simulink model "SPGF_FSK_0000_R2022b"  (R2022b)
settings: Solver=ode4  StartTime=0.0  StopTime=1.4  FixedStep=50e-6/50  RelTol=1e-3  EnableMultiTasking=on
undefined symbols (not defined in the file): D11, Delta
libraries: spsSeriesRLCBranchLib x1646, spsGroundLib x360, spsStairGeneratorLib x147, spsIdealSwitchLib x145, spsCurrentMeasurementLib x145, spsUniversalBridgeLib x76, spsThreePhaseSeriesRLCLoadLib x57, simulink x45, spsBistableLib x36, spsSequenceAnalyzerLib x31, spsThreePhaseParallelRLCLoadLib x20, spsThreePhaseTransformerTwoWindingsLib x20
(part 6 of 40)

== system SPGF_FSK_0000_R2022b/TP42 ==
  Load : spsThreePhaseParallelRLCLoadLib/Three-Phase Parallel RLC Load  Commented=on  LConnTagsString=A|B|C  Configuration=Y (grounded)  NominalVoltage=380  Vabc=[1e3 1e3 1e3]  Vabcp=[1e3 1e3 1e3]  NominalFrequency=50  UnbalancedPower=off  ActivePower=352800  InductivePower=158760  CapacitivePower=0  Pabc=[10e3 9e3 11e3]  QLabc=[100 90 110]  QCabc=[100 90 110]  Pabcp=[10e3 9e3 11e3]  QLabcp=[100 90 110]  QCabcp=[100 90 110]  Measurements=None  LoadType=constant PQ
  Nonlinear Load : Subsystem  Commented=on
  Nonlinear Load 3ph : Subsystem
  Q : Subsystem
  T : spsThreePhaseTransformerTwoWindingsLib/Three-Phase Transformer (Two Windings)  Winding1Connection=Delta (D11)  Winding2Connection=Yg  CoreType=Three single-phase transformers  SetSaturation=on  Hysteresis=off  DataFile='hysteresis'  SetInitialFlux=off  Measurements=None  UNITS=pu  NominalPower=[630000, 50]  Winding1=[10250, 0.00603175, 0.02750000]  Winding2=[400.00, 0.00603175, 0.02750000]  Rm=504  Lm=58.8235  L0=2  Saturation=[0 0;0.01774 0.324129;0.0487637 0.61284;0.0980856 0.825118;0.2 1;0.309543 1.08024;0.652348 1.17344;2.0357 1.26115;6.0215 1.36094;12.4388 1.49469]  InitialFluxes=[0.547022493837308 0.502268865215099 -1.04929135905267]  BreakLoop=on  DiscreteSolver=Trapezoidal iterative  DataType=off  TransfoNumber=1
  Three-Phase Series RLC Load : spsThreePhaseSeriesRLCLoadLib/Three-Phase Series RLC Load  Commented=on  LConnTagsString=A|B|C  Configuration=Y (grounded)  NominalVoltage=380  Vabc=[1e3 1e3 1e3]  Vabcp=[1e3 1e3 1e3]  NominalFrequency=50  UnbalancedPower=off  ActivePower=352800  InductivePower=158760  CapacitivePower=0  Pabc=[10e3 9e3 11e3]  QLabc=[100 90 110]  QCabc=[100 90 110]  Pabcp=[10e3 9e3 11e3]  QLabcp=[100 90 110]  QCabcp=[100 90 110]  Measurements=None  LoadType=constant Z
  Three-Phase Series RLC Load1 : spsThreePhaseSeriesRLCLoadLib/Three-Phase Series RLC Load  LConnTagsString=A|B|C  Configuration=Y (grounded)  NominalVoltage=380  Vabc=[1e3 1e3 1e3]  Vabcp=[1e3 1e3 1e3]  NominalFrequency=50  UnbalancedPower=off  ActivePower=0.1*352800  InductivePower=0  CapacitivePower=0  Pabc=[10e3 9e3 11e3]  QLabc=[100 90 110]  QCabc=[100 90 110]  Pabcp=[10e3 9e3 11e3]  QLabcp=[100 90 110]  QCabcp=[100 90 110]  Measurements=None  LoadType=constant Z
  Three-Phase Series RLC Load2 : spsThreePhaseSeriesRLCLoadLib/Three-Phase Series RLC Load  LConnTagsString=A|B|C  Configuration=Y (grounded)  NominalVoltage=380  Vabc=[1e3 1e3 1e3]  Vabcp=[1e3 1e3 1e3]  NominalFrequency=50  UnbalancedPower=off  ActivePower=0.9*352800  InductivePower=158760  CapacitivePower=0  Pabc=[10e3 9e3 11e3]  QLabc=[100 90 110]  QCabc=[100 90 110]  Pabcp=[10e3 9e3 11e3]  QLabcp=[100 90 110]  QCabcp=[100 90 110]  Measurements=None  LoadType=constant Z
  A : PMIOPort  Side=Right
  B : PMIOPort  Port=2  Side=Right
  C : PMIOPort  Port=3  Side=Right
  connections:
  Q/LConn3 -- T/LConn3
  Q/LConn1 -- T/LConn1
  Q/RConn2 -- B/RConn1
  Q/RConn1 -- A/RConn1
  Q/LConn2 -- T/LConn2
  Q/RConn3 -- C/RConn1
  Three-Phase Series RLC Load1/LConn3 -- Three-Phase Series RLC Load2/LConn3 -- Three-Phase Series RLC Load/LConn3 -- Nonlinear Load/LConn3 -- Nonlinear Load 3ph/LConn3 -- T/RConn3 -- Load/LConn3
  Three-Phase Series RLC Load1/LConn2 -- Three-Phase Series RLC Load2/LConn2 -- Three-Phase Series RLC Load/LConn2 -- Nonlinear Load/LConn2 -- Nonlinear Load 3ph/LConn2 -- Load/LConn2 -- T/RConn2
  Three-Phase Series RLC Load2/LConn1 -- Three-Phase Series RLC Load1/LConn1 -- Three-Phase Series RLC Load/LConn1 -- Nonlinear Load/LConn1 -- Nonlinear Load 3ph/LConn1 -- Load/LConn1 -- T/RConn1

== system SPGF_FSK_0000_R2022b/TP43 ==
  Load : spsThreePhaseParallelRLCLoadLib/Three-Phase Parallel RLC Load  Commented=on  LConnTagsString=A|B|C  Configuration=Y (grounded)  NominalVoltage=380  Vabc=[1e3 1e3 1e3]  Vabcp=[1e3 1e3 1e3]  NominalFrequency=50  UnbalancedPower=off  ActivePower=224000  InductivePower=100800  CapacitivePower=0  Pabc=[10e3 9e3 11e3]  QLabc=[100 90 110]  QCabc=[100 90 110]  Pabcp=[10e3 9e3 11e3]  QLabcp=[100 90 110]  QCabcp=[100 90 110]  Measurements=None  LoadType=constant PQ
  Nonlinear Load : Subsystem  Commented=on
  Nonlinear Load 3ph : Subsystem
  Q : Subsystem
  T : spsThreePhaseTransformerTwoWindingsLib/Three-Phase Transformer (Two Windings)  Winding1Connection=Y  Winding2Connection=Yg  CoreType=Three single-phase transformers  SetSaturation=on  Hysteresis=off  DataFile='hysteresis'  SetInitialFlux=off  Measurements=None  UNITS=pu  NominalPower=[400000, 50]  Winding1=[10250, 0.00687500, 0.02250000]  Winding2=[400.00, 0.00687500, 0.02250000]  Rm=444.444  Lm=55.5556  L0=2  Saturation=[0 0;0.01774 0.324129;0.0487637 0.61284;0.0980856 0.825118;0.2 1;0.309543 1.08024;0.652348 1.17344;2.0357 1.26115;6.0215 1.36094;12.4388 1.49469]  InitialFluxes=[0.0224556996451499 0.89821690421441 -0.920672603859515]  BreakLoop=on  DiscreteSolver=Trapezoidal iterative  DataType=off  TransfoNumber=1
  Three-Phase Series RLC Load : spsThreePhaseSeriesRLCLoadLib/Three-Phase Series RLC Load  Commented=on  LConnTagsString=A|B|C  Configuration=Y (grounded)  NominalVoltage=380  Vabc=[1e3 1e3 1e3]  Vabcp=[1e3 1e3 1e3]  NominalFrequency=50  UnbalancedPower=off  ActivePower=224000  InductivePower=100800  CapacitivePower=0  Pabc=[10e3 9e3 11e3]  QLabc=[100 90 110]  QCabc=[100 90 110]  Pabcp=[10e3 9e3 11e3]  QLabcp=[100 90 110]  QCabcp=[100 90 110]  Measurements=None  LoadType=constant Z
  Three-Phase Series RLC Load1 : spsThreePhaseSeriesRLCLoadLib/Three-Phase Series RLC Load  LConnTagsString=A|B|C  Configuration=Y (grounded)  NominalVoltage=380  Vabc=[1e3 1e3 1e3]  Vabcp=[1e3 1e3 1e3]  NominalFrequency=50  UnbalancedPower=off  ActivePower=0.1*224000  InductivePower=0  CapacitivePower=0  Pabc=[10e3 9e3 11e3]  QLabc=[100 90 110]  QCabc=[100 90 110]  Pabcp=[10e3 9e3 11e3]  QLabcp=[100 90 110]  QCabcp=[100 90 110]  Measurements=None  LoadType=constant Z
  Three-Phase Series RLC Load2 : spsThreePhaseSeriesRLCLoadLib/Three-Phase Series RLC Load  LConnTagsString=A|B|C  Configuration=Y (grounded)  NominalVoltage=380  Vabc=[1e3 1e3 1e3]  Vabcp=[1e3 1e3 1e3]  NominalFrequency=50  UnbalancedPower=off  ActivePower=0.9*224000  InductivePower=100800  CapacitivePower=0  Pabc=[10e3 9e3 11e3]  QLabc=[100 90 110]  QCabc=[100 90 110]  Pabcp=[10e3 9e3 11e3]  QLabcp=[100 90 110]  QCabcp=[100 90 110]  Measurements=None  LoadType=constant Z
  A : PMIOPort  Side=Right
  B : PMIOPort  Port=2  Side=Right
  C : PMIOPort  Port=3  Side=Right
  connections:
  Three-Phase Series RLC Load2/LConn1 -- Three-Phase Series RLC Load1/LConn1 -- Three-Phase Series RLC Load/LConn1 -- Nonlinear Load/LConn1 -- Nonlinear Load 3ph/LConn1 -- Load/LConn1 -- T/RConn1
  Three-Phase Series RLC Load2/LConn2 -- Three-Phase Series RLC Load1/LConn2 -- Three-Phase Series RLC Load/LConn2 -- Nonlinear Load/LConn2 -- Nonlinear Load 3ph/LConn2 -- Load/LConn2 -- T/RConn2
  Three-Phase Series RLC Load2/LConn3 -- Three-Phase Series RLC Load1/LConn3 -- Three-Phase Series RLC Load/LConn3 -- Nonlinear Load/LConn3 -- Nonlinear Load 3ph/LConn3 -- T/RConn3 -- Load/LConn3
  Q/RConn3 -- C/RConn1
  Q/LConn2 -- T/LConn2
  Q/RConn1 -- A/RConn1
  Q/RConn2 -- B/RConn1
  Q/LConn1 -- T/LConn1
  Q/LConn3 -- T/LConn3

== system SPGF_FSK_0000_R2022b/TP51 ==
  Load : spsThreePhaseParallelRLCLoadLib/Three-Phase Parallel RLC Load  Commented=on  LConnTagsString=A|B|C  Configuration=Y (grounded)  NominalVoltage=380  Vabc=[1e3 1e3 1e3]  Vabcp=[1e3 1e3 1e3]  NominalFrequency=50  UnbalancedPower=off  ActivePower=224000  InductivePower=100800  CapacitivePower=0  Pabc=[10e3 9e3 11e3]  QLabc=[100 90 110]  QCabc=[100 90 110]  Pabcp=[10e3 9e3 11e3]  QLabcp=[100 90 110]  QCabcp=[100 90 110]  Measurements=None  LoadType=constant PQ
  Nonlinear Load : Subsystem  Commented=on
  Nonlinear Load 3ph : Subsystem
  Q : Subsystem
  T : spsThreePhaseTransformerTwoWindingsLib/Three-Phase Transformer (Two Windings)  Winding1Connection=Y  Winding2Connection=Yg  CoreType=Three single-phase transformers  SetSaturation=on  Hysteresis=off  DataFile='hysteresis'  SetInitialFlux=off  Measurements=None  UNITS=pu  NominalPower=[400000, 50]  Winding1=[10250, 0.00687500, 0.02250000]  Winding2=[400.00, 0.00687500, 0.02250000]  Rm=444.444  Lm=55.5556  L0=2  Saturation=[0 0;0.01774 0.324129;0.0487637 0.61284;0.0980856 0.825118;0.2 1;0.309543 1.08024;0.652348 1.17344;2.0357 1.26115;6.0215 1.36094;12.4388 1.49469]  InitialFluxes=[0.0226319899806227 0.898092550893289 -0.920724540873739]  BreakLoop=on  DiscreteSolver=Trapezoidal iterative  DataType=off  TransfoNumber=1
  Three-Phase Series RLC Load : spsThreePhaseSeriesRLCLoadLib/Three-Phase Series RLC Load  Commented=on  LConnTagsString=A|B|C  Configuration=Y (grounded)  NominalVoltage=380  Vabc=[1e3 1e3 1e3]  Vabcp=[1e3 1e3 1e3]  NominalFrequency=50  UnbalancedPower=off  ActivePower=224000  InductivePower=100800  CapacitivePower=0  Pabc=[10e3 9e3 11e3]  QLabc=[100 90 110]  QCabc=[100 90 110]  Pabcp=[10e3 9e3 11e3]  QLabcp=[100 90 110]  QCabcp=[100 90 110]  Measurements=None  LoadType=constant Z
  Three-Phase Series RLC Load1 : spsThreePhaseSeriesRLCLoadLib/Three-Phase Series RLC Load  LConnTagsString=A|B|C  Configuration=Y (grounded)  NominalVoltage=380  Vabc=[1e3 1e3 1e3]  Vabcp=[1e3 1e3 1e3]  NominalFrequency=50  UnbalancedPower=off  ActivePower=0.1*224000  InductivePower=0  CapacitivePower=0  Pabc=[10e3 9e3 11e3]  QLabc=[100 90 110]  QCabc=[100 90 110]  Pabcp=[10e3 9e3 11e3]  QLabcp=[100 90 110]  QCabcp=[100 90 110]  Measurements=None  LoadType=constant Z
  Three-Phase Series RLC Load2 : spsThreePhaseSeriesRLCLoadLib/Three-Phase Series RLC Load  LConnTagsString=A|B|C  Configuration=Y (grounded)  NominalVoltage=380  Vabc=[1e3 1e3 1e3]  Vabcp=[1e3 1e3 1e3]  NominalFrequency=50  UnbalancedPower=off  ActivePower=0.9*224000  InductivePower=100800  CapacitivePower=0  Pabc=[10e3 9e3 11e3]  QLabc=[100 90 110]  QCabc=[100 90 110]  Pabcp=[10e3 9e3 11e3]  QLabcp=[100 90 110]  QCabcp=[100 90 110]  Measurements=None  LoadType=constant Z
  A : PMIOPort  Side=Right
  B : PMIOPort  Port=2  Side=Right
  C : PMIOPort  Port=3  Side=Right
  connections:
  Three-Phase Series RLC Load2/LConn1 -- Three-Phase Series RLC Load1/LConn1 -- Three-Phase Series RLC Load/LConn1 -- Nonlinear Load/LConn1 -- Nonlinear Load 3ph/LConn1 -- Load/LConn1 -- T/RConn1
  Three-Phase Series RLC Load2/LConn2 -- Three-Phase Series RLC Load1/LConn2 -- Three-Phase Series RLC Load/LConn2 -- Nonlinear Load/LConn2 -- Nonlinear Load 3ph/LConn2 -- Load/LConn2 -- T/RConn2
  Three-Phase Series RLC Load1/LConn3 -- Three-Phase Series RLC Load2/LConn3 -- Three-Phase Series RLC Load/LConn3 -- Nonlinear Load/LConn3 -- Nonlinear Load 3ph/LConn3 -- T/RConn3 -- Load/LConn3
  Q/RConn3 -- C/RConn1
  Q/LConn2 -- T/LConn2
  Q/RConn1 -- A/RConn1
  Q/RConn2 -- B/RConn1
  Q/LConn1 -- T/LConn1
  Q/LConn3 -- T/LConn3

== system SPGF_FSK_0000_R2022b/TP52 ==
  Load : spsThreePhaseParallelRLCLoadLib/Three-Phase Parallel RLC Load  Commented=on  LConnTagsString=A|B|C  Configuration=Y (grounded)  NominalVoltage=380  Vabc=[1e3 1e3 1e3]  Vabcp=[1e3 1e3 1e3]  NominalFrequency=50  UnbalancedPower=off  ActivePower=560000  InductivePower=252000  CapacitivePower=0  Pabc=[10e3 9e3 11e3]  QLabc=[100 90 110]  QCabc=[100 90 110]  Pabcp=[10e3 9e3 11e3]  QLabcp=[100 90 110]  QCabcp=[100 90 110]  Measurements=None  LoadType=constant PQ
  Nonlinear Load : Subsystem  Commented=on
  Nonlinear Load 3ph : Subsystem
  Q : Subsystem
  T : spsThreePhaseTransformerTwoWindingsLib/Three-Phase Transformer (Two Windings)  Winding1Connection=Y  Winding2Connection=Yg  CoreType=Three single-phase transformers  SetSaturation=on  Hysteresis=off  DataFile='hysteresis'  SetInitialFlux=off  Measurements=None  UNITS=pu  NominalPower=[1000000, 50]  Winding1=[10250, 0.00610000, 0.02750000]  Winding2=[400.00, 0.00610000, 0.02750000]  Rm=526.316  Lm=58.8235  L0=2  Saturation=[0 0;0.01774 0.324129;0.0487637 0.61284;0.0980856 0.825118;0.2 1;0.309543 1.08024;0.652348 1.17344;2.0357 1.26115;6.0215 1.36094;12.4388 1.49469]  InitialFluxes=[0.0255116004445126 0.893899314027236 -0.919410914471723]  BreakLoop=on  DiscreteSolver=Trapezoidal iterative  DataType=off  TransfoNumber=1
  Three-Phase Series RLC Load : spsThreePhaseSeriesRLCLoadLib/Three-Phase Series RLC Load  Commented=on  LConnTagsString=A|B|C  Configuration=Y (grounded)  NominalVoltage=380  Vabc=[1e3 1e3 1e3]  Vabcp=[1e3 1e3 1e3]  NominalFrequency=50  UnbalancedPower=off  ActivePower=560000  InductivePower=252000  CapacitivePower=0  Pabc=[10e3 9e3 11e3]  QLabc=[100 90 110]  QCabc=[100 90 110]  Pabcp=[10e3 9e3 11e3]  QLabcp=[100 90 110]  QCabcp=[100 90 110]  Measurements=None  LoadType=constant Z
  Three-Phase Series RLC Load1 : spsThreePhaseSeriesRLCLoadLib/Three-Phase Series RLC Load  LConnTagsString=A|B|C  Configuration=Y (grounded)  NominalVoltage=380  Vabc=[1e3 1e3 1e3]  Vabcp=[1e3 1e3 1e3]  NominalFrequency=50  UnbalancedPower=off  ActivePower=0.1*560000  InductivePower=0  CapacitivePower=0  Pabc=[10e3 9e3 11e3]  QLabc=[100 90 110]  QCabc=[100 90 110]  Pabcp=[10e3 9e3 11e3]  QLabcp=[100 90 110]  QCabcp=[100 90 110]  Measurements=None  LoadType=constant Z
  Three-Phase Series RLC Load2 : spsThreePhaseSeriesRLCLoadLib/Three-Phase Series RLC Load  LConnTagsString=A|B|C  Configuration=Y (grounded)  NominalVoltage=380  Vabc=[1e3 1e3 1e3]  Vabcp=[1e3 1e3 1e3]  NominalFrequency=50  UnbalancedPower=off  ActivePower=0.9*560000  InductivePower=252000  CapacitivePower=0  Pabc=[10e3 9e3 11e3]  QLabc=[100 90 110]  QCabc=[100 90 110]  Pabcp=[10e3 9e3 11e3]  QLabcp=[100 90 110]  QCabcp=[100 90 110]  Measurements=None  LoadType=constant Z
  A : PMIOPort  Side=Right
  B : PMIOPort  Port=2  Side=Right
  C : PMIOPort  Port=3  Side=Right
  connections:
  Q/LConn3 -- T/LConn3
  Q/LConn1 -- T/LConn1
  Q/RConn2 -- B/RConn1
  Q/RConn1 -- A/RConn1
  Q/LConn2 -- T/LConn2
  Q/RConn3 -- C/RConn1
  Three-Phase Series RLC Load1/LConn3 -- Three-Phase Series RLC Load2/LConn3 -- Nonlinear Load/LConn3 -- Nonlinear Load 3ph/LConn3 -- T/RConn3 -- Load/LConn3 -- Three-Phase Series RLC Load/LConn3
  Three-Phase Series RLC Load1/LConn2 -- Three-Phase Series RLC Load2/LConn2 -- Nonlinear Load/LConn2 -- Nonlinear Load 3ph/LConn2 -- Load/LConn2 -- T/RConn2 -- Three-Phase Series RLC Load/LConn2
  Three-Phase Series RLC Load/LConn1 -- Nonlinear Load/LConn1 -- Nonlinear Load 3ph/LConn1 -- T/RConn1 -- Load/LConn1 -- Three-Phase Series RLC Load2/LConn1 -- Three-Phase Series RLC Load1/LConn1

== system SPGF_FSK_0000_R2022b/TP53 ==
  Load : spsThreePhaseParallelRLCLoadLib/Three-Phase Parallel RLC Load  Commented=on  LConnTagsString=A|B|C  Configuration=Y (grounded)  NominalVoltage=380  Vabc=[1e3 1e3 1e3]  Vabcp=[1e3 1e3 1e3]  NominalFrequency=50  UnbalancedPower=off  ActivePower=224000  InductivePower=100800  CapacitivePower=0  Pabc=[10e3 9e3 11e3]  QLabc=[100 90 110]  QCabc=[100 90 110]  Pabcp=[10e3 9e3 11e3]  QLabcp=[100 90 110]  QCabcp=[100 90 110]  Measurements=None  LoadType=constant PQ
  Nonlinear Load : Subsystem  Commented=on
  Nonlinear Load 3ph : Subsystem
  Q : Subsystem
  T : spsThreePhaseTransformerTwoWindingsLib/Three-Phase Transformer (Two Windings)  Winding1Connection=Y  Winding2Connection=Yg  CoreType=Three single-phase transformers  SetSaturation=on  Hysteresis=off  DataFile='hysteresis'  SetInitialFlux=off  Measurements=None  UNITS=pu  NominalPower=[400000, 50]  Winding1=[10250, 0.00687500, 0.02250000]  Winding2=[400.00, 0.00687500, 0.02250000]  Rm=444.444  Lm=55.5556  L0=2  Saturation=[0 0;0.01774 0.324129;0.0487637 0.61284;0.0980856 0.825118;0.2 1;0.309543 1.08024;0.652348 1.17344;2.0357 1.26115;6.0215 1.36094;12.4388 1.49469]  InitialFluxes=[0.0221773071271057 0.896403452288866 -0.918580759415872]  BreakLoop=on  DiscreteSolver=Trapezoidal iterative  DataType=off  TransfoNumber=1
  Three-Phase Series RLC Load : spsThreePhaseSeriesRLCLoadLib/Three-Phase Series RLC Load  Commented=on  LConnTagsString=A|B|C  Configuration=Y (grounded)  NominalVoltage=380  Vabc=[1e3 1e3 1e3]  Vabcp=[1e3 1e3 1e3]  NominalFrequency=50  UnbalancedPower=off  ActivePower=224000  InductivePower=100800  CapacitivePower=0  Pabc=[10e3 9e3 11e3]  QLabc=[100 90 110]  QCabc=[100 90 110]  Pabcp=[10e3 9e3 11e3]  QLabcp=[100 90 110]  QCabcp=[100 90 110]  Measurements=None  LoadType=constant Z
  Three-Phase Series RLC Load1 : spsThreePhaseSeriesRLCLoadLib/Three-Phase Series RLC Load  LConnTagsString=A|B|C  Configuration=Y (grounded)  NominalVoltage=380  Vabc=[1e3 1e3 1e3]  Vabcp=[1e3 1e3 1e3]  NominalFrequency=50  UnbalancedPower=off  ActivePower=0.1*224000  InductivePower=0  CapacitivePower=0  Pabc=[10e3 9e3 11e3]  QLabc=[100 90 110]  QCabc=[100 90 110]  Pabcp=[10e3 9e3 11e3]  QLabcp=[100 90 110]  QCabcp=[100 90 110]  Measurements=None  LoadType=constant Z
  Three-Phase Series RLC Load2 : spsThreePhaseSeriesRLCLoadLib/Three-Phase Series RLC Load  LConnTagsString=A|B|C  Configuration=Y (grounded)  NominalVoltage=380  Vabc=[1e3 1e3 1e3]  Vabcp=[1e3 1e3 1e3]  NominalFrequency=50  UnbalancedPower=off  ActivePower=0.9*224000  InductivePower=100800  CapacitivePower=0  Pabc=[10e3 9e3 11e3]  QLabc=[100 90 110]  QCabc=[100 90 110]  Pabcp=[10e3 9e3 11e3]  QLabcp=[100 90 110]  QCabcp=[100 90 110]  Measurements=None  LoadType=constant Z
  A : PMIOPort  Side=Right
  B : PMIOPort  Port=2  Side=Right
  C : PMIOPort  Port=3  Side=Right
  connections:
  Three-Phase Series RLC Load1/LConn1 -- Three-Phase Series RLC Load2/LConn1 -- Three-Phase Series RLC Load/LConn1 -- Nonlinear Load/LConn1 -- Nonlinear Load 3ph/LConn1 -- T/RConn1 -- Load/LConn1
  Three-Phase Series RLC Load2/LConn2 -- Three-Phase Series RLC Load1/LConn2 -- Three-Phase Series RLC Load/LConn2 -- Nonlinear Load/LConn2 -- Nonlinear Load 3ph/LConn2 -- T/RConn2 -- Load/LConn2
  Three-Phase Series RLC Load2/LConn3 -- Three-Phase Series RLC Load1/LConn3 -- Three-Phase Series RLC Load/LConn3 -- Nonlinear Load/LConn3 -- Nonlinear Load 3ph/LConn3 -- T/RConn3 -- Load/LConn3
  Q/RConn3 -- C/RConn1
  Q/LConn2 -- T/LConn2
  Q/RConn1 -- A/RConn1
  Q/RConn2 -- B/RConn1
  Q/LConn1 -- T/LConn1
  Q/LConn3 -- T/LConn3

== system SPGF_FSK_0000_R2022b/TSN ==
  DGR : Subsystem  Commented=on  mask{Freq=50, Current=19.26, CompFactor=0, Voltage=6090, Lt=0.0091667, TangLoss=0.02}
      mask prompts: Freq "Frequency, [Hz]"; Current "Compensated Current, [A]"; CompFactor "Compensation Factor, [-0.2,..., 0.2]"; Voltage "Voltage at DGR"; Lt "Transformer inductance [ L1(H)]"; TangLoss "Loss factor"
      mask init:
      | % L = 1350e-3;
      | Icomp = -(CompFactor*Current-Current);
      | L = (Voltage/Icomp)/(2*pi*Freq)-Lt;
      | Rm = 2*pi*Freq*L*TangLoss/2;
      | Rst = ((2*pi*Freq*L)^2+Rm^2)/Rm;
  Ground1 : spsGroundLib/Ground  Commented=on  LConnTagsString=a
  Rst : spsSeriesRLCBranchLib/Series RLC Branch  Commented=on  LConnTagsString=__new0  RConnTagsString=__new0  BranchType=R  Resistance=100  Inductance=1000e-3  SetiL0=off  InitialCurrent=0  Capacitance=1e-6  Setx0=off  InitialVoltage=0  Measurements=None
  TSN : spsThreePhaseTransformerTwoWindingsLib/Three-Phase Transformer (Two Windings)  Winding1Connection=Yn  Winding2Connection=Delta (D11)  CoreType=Three single-phase transformers  SetSaturation=on  Hysteresis=off  DataFile='hysteresis'  SetInitialFlux=off  Measurements=None  UNITS=pu  NominalPower=[250000 50]  Winding1=[10250 0.0076 0.0275]  Winding2=[400 0.0076 0.0275]  Rm=249.99  Lm=28.571  L0=0.66885  Saturation=[0 0;0.0010988 0.1;0.0024217 0.2;0.0040219 0.3;0.0059961 0.40001;0.0084933 0.50001;0.011751 0.60001;0.016177 0.70001;0.022532 0.80001;0.032408 0.90001;0.049756 1;0.087393 1.1;0.20927 1.2;0.70928 1.3;1.5874 1.4;2.5497 1.5]  InitialFluxes=[0.0107246931876914 0.916304027052604 -0.927028720240254]  BreakLoop=on  DiscreteSolver=Trapezoidal iterative  DataType=off  TransfoNumber=1
  A : PMIOPort  Side=Left
  B : PMIOPort  Port=2  Side=Left
  C : PMIOPort  Port=3  Side=Left
  connections:
  TSN/LConn1 -- A/RConn1
  TSN/LConn3 -- C/RConn1
  TSN/LConn2 -- B/RConn1
  DGR/RConn1 -- Rst/RConn1 -- TSN/LConn4
  Ground1/LConn1 -- Rst/LConn1

== system SPGF_FSK_0000_R2022b/V1 ==
  Sum of Elements : Sum  Inputs=+
  Three-Phase V-I Measurement : spsThreePhaseVIMeasurementLib/Three-Phase V-I Measurement  VoltageMeasurement=phase-to-ground  SetLabelV=off  LabelV=Vabc  Vpu=off  VpuLL=off  CurrentMeasurement=no  SetLabelI=off  LabelI=Iabc  Ipu=off  Pbase=100e6  Vbase=500e3  OutputType=Complex  PhasorSimulation=off  PSBequivalent=0
  VT : Subsystem
  A : PMIOPort  Side=Left
  B : PMIOPort  Port=2  Side=Left
  C : PMIOPort  Port=3  Side=Left
  tag scope: M3U0_V1=global, M3U0_VT1=global, MUabc1_VT1=global, MUabc2_VT1=global, MUabc_V1=global
  wires:
  VT/1(Uabc1) -> [MUabc1_VT1]
  VT/2(Uabc2) -> [MUabc2_VT1]
  VT/3(3U0) -> [M3U0_VT1]
  Sum of Elements/1 -> [M3U0_V1]
  Three-Phase V-I Measurement/1 -> [MUabc_V1], Sum of Elements/1
  connections:
  VT/LConn2 -- Three-Phase V-I Measurement/LConn2 -- B/RConn1
  Three-Phase V-I Measurement/LConn1 -- VT/LConn1 -- A/RConn1
  C/RConn1 -- Three-Phase V-I Measurement/LConn3 -- VT/LConn3

== system SPGF_FSK_0000_R2022b/V53 ==
  VT : Subsystem
  A : PMIOPort  Side=Left
  B : PMIOPort  Port=2  Side=Left
  C : PMIOPort  Port=3  Side=Left
  tag scope: M3U0_VT53=global, MUabc1_VT53=global, MUabc2_VT53=global
  wires:
  VT/1(Uabc1) -> [MUabc1_VT53]
  VT/2(Uabc2) -> [MUabc2_VT53]
  VT/3(3U0) -> [M3U0_VT53]
  connections:
  VT/LConn2 -- B/RConn1
  VT/LConn1 -- A/RConn1
  VT/LConn3 -- C/RConn1

== system SPGF_FSK_0000_R2022b/W11 ==
  DPL : Subsystem  Commented=on  mask{N=6, Frequency=[50], R_matrix=[0.16804171053251 0.0494303508468275 0.0494307138863892 0.0494307138863892 0.0494307138863892 0.0494307138863892;0.0494303508468275 0.453964608408466 0.0494307138863892 0.0494307138863892 0.0494307138863892 0.0494307138863892;0.0494307138863892 0.0494307138863892 0.168042542894219 0.0494311832085362 0.0494315463631826 0.0494315463631826;0.0494307138863892 0.0494307138863892 0.0494311832085362 0.453965440770175 0.0494315463631826 0.0494315463631826;0.0494307138863892 0.0494307138863892 0.0494315463631826 0.0494315463631826 0.168042542894219 0.0494311832085362;0.0494307138863892 0.0494307138863892 0.0494315463631826 0.0494315463631826 0.0494311832085362 0.453965440770175], L_matrix=[0.00251009633073536 0.00236486393083554 0.00216527915989806 0.00216527915989806 0.00216527915989806 0.00216527915989806;0.00236486393083554 0.00236372630589008 0.00216527915989806 0.00216527915989806 0.00216527915989806 0.00216527915989806;0.00216527915989806 0.00216527915989806 0.00243730728151529 0.00229207488161547 0.00218759083544916 0.00218759083544916;0.00216527915989806 0.00216527915989806 0.00229207488161547 0.00229093725667002 0.00218759083544916 0.00218759083544916;0.00216527915989806 0.00216527915989806 0.00218759083544916 0.00218759083544916 0.00243730728151529 0.00229207488161547;0.00216527915989806 0.00216527915989806 0.00218759083544916 0.00218759083544916 0.00229207488161547 0.00229093725667002], C_matrix=[2.72330746828679e-07 -2.72330746828679e-07 0 0 0 0;-2.72330746828679e-07 4.53349993591203e-07 0 0 0 0;0 0 2.72330746828679e-07 -2.72330746828679e-07 0 0;0 0 -2.72330746828679e-07 4.53349993591203e-07 0 0;0 0 0 0 2.72330746828679e-07 -2.72330746828679e-07;0 0 0 0 -2.72330746828679e-07 4.53349993591203e-07], Rg_matrix=[584417.826283929 -584417.826283929 Inf Inf Inf -Inf;-584417.826283929 351064.178541512 Inf Inf Inf -Inf;Inf Inf 584417.826283929 -584417.826283929 Inf -Inf;Inf Inf -584417.826283929 351064.178541512 Inf -Inf;Inf Inf Inf Inf 584417.826283929 -584417.826283929;Inf Inf Inf Inf -584417.826283929 351064.178541512], LineLength=[3]}
      mask prompts: N "Number of phases [N]"; Frequency "Frequency used for rlc specification [Hz]:"; R_matrix "Resistance per unit length [Ohms/km] NxN matrix"; L_matrix "Inductance per unit length [H/km] NxN matrix"; C_matrix "Capacitance per unit length [F/km] NxN matrix"; Rg_matrix "Resistance shunt matrix 6*6 [Ohm*km]"; LineLength "Line Length(km)"
      mask init:
      | % Rloss=1/(2*pi*Frequency*C_matrix(1,1)*TangLoss);
      | Rg_matrix=Rg_matrix./LineLength;
      mask Display:
      | port_label('lconn',1,'A');
      | port_label('lconn',2,'B');
      | port_label('lconn',3,'C');
      | 
      | port_label('rconn',1,'a');
      | port_label('rconn',2,'b');
      | port_label('rconn',3,'c');
      | 
      | disp('1x240');
  Pi : Subsystem  mask{R0=0.125, X0=0.075, Cp0=0.46, tg=2, Frequency=[50], LineLength=[3]}
      mask prompts: R0 "Удельное активное сопротивление, Ом/км"; X0 "Удельное индуктивное сопротивление, Ом/км"; Cp0 "Удельная рабочая емкость, мкФ/км"; tg "Тангенс диэлектрических потерь, %"; Frequency "Частота сети, Гц"; LineLength "Длина линии, км"
      mask init:
      | R=R0*LineLength;
      | L=X0*LineLength/(2*pi*Frequency);
      | Cp=Cp0*LineLength*1e-6;
      | Cmf=0.1525*Cp;
      | Cfg=0.56*Cp;
      | tg_pu=tg/100;
      | 
      | Rmf=1/(Cmf*2*pi*Frequency*tg_pu);
      | Rfg=1/(Cfg*2*pi*Frequency*tg_pu);
      mask Display:
      | port_label('lconn',1,'A');
      | port_label('lconn',2,'B');
      | port_label('lconn',3,'C');
      | 
      | port_label('rconn',1,'a');
      | port_label('rconn',2,'b');
      | port_label('rconn',3,'c');
      | 
      | disp('1x240');
  Q : Subsystem
  concentrated : Subsystem  Commented=on  mask{N=6, Frequency=[50], R_matrix=[0.16804171053251 0.0494303508468275 0.0494307138863892 0.0494307138863892 0.0494307138863892 0.0494307138863892;0.0494303508468275 0.453964608408466 0.0494307138863892 0.0494307138863892 0.0494307138863892 0.0494307138863892;0.0494307138863892 0.0494307138863892 0.168042542894219 0.0494311832085362 0.0494315463631826 0.0494315463631826;0.0494307138863892 0.0494307138863892 0.0494311832085362 0.453965440770175 0.0494315463631826 0.0494315463631826;0.0494307138863892 0.0494307138863892 0.0494315463631826 0.0494315463631826 0.168042542894219 0.0494311832085362;0.0494307138863892 0.0494307138863892 0.0494315463631826 0.0494315463631826 0.0494311832085362 0.453965440770175], L_matrix=[0.00251009633073536 0.00236486393083554 0.00216527915989806 0.00216527915989806 0.00216527915989806 0.00216527915989806;0.00236486393083554 0.00236372630589008 0.00216527915989806 0.00216527915989806 0.00216527915989806 0.00216527915989806;0.00216527915989806 0.00216527915989806 0.00243730728151529 0.00229207488161547 0.00218759083544916 0.00218759083544916;0.00216527915989806 0.00216527915989806 0.00229207488161547 0.00229093725667002 0.00218759083544916 0.00218759083544916;0.00216527915989806 0.00216527915989806 0.00218759083544916 0.00218759083544916 0.00243730728151529 0.00229207488161547;0.00216527915989806 0.00216527915989806 0.00218759083544916 0.00218759083544916 0.00229207488161547 0.00229093725667002], C_matrix=[2.72330746828679e-07 -2.72330746828679e-07 0 0 0 0;-2.72330746828679e-07 4.53349993591203e-07 0 0 0 0;0 0 2.72330746828679e-07 -2.72330746828679e-07 0 0;0 0 -2.72330746828679e-07 4.53349993591203e-07 0 0;0 0 0 0 2.72330746828679e-07 -2.72330746828679e-07;0 0 0 0 -2.72330746828679e-07 4.53349993591203e-07], Rg_matrix=[584417.826283929 -584417.826283929 Inf Inf Inf -Inf;-584417.826283929 351064.178541512 Inf Inf Inf -Inf;Inf Inf 584417.826283929 -584417.826283929 Inf -Inf;Inf Inf -584417.826283929 351064.178541512 Inf -Inf;Inf Inf Inf Inf 584417.826283929 -584417.826283929;Inf Inf Inf Inf -584417.826283929 351064.178541512], LineLength=[3]}
      mask prompts: N "Number of phases [N]"; Frequency "Frequency [Hz]:"; R_matrix "Resistance matrix 6*6 [Ohm/km]"; L_matrix "Inductance matrix 6*6 [H/km]"; C_matrix "Capacitance matrix 6*6 [F/km]"; Rg_matrix "Resistance shunt matrix 6*6 [Ohm*km]"; LineLength "Line Length(km)"
      mask init:
      | R_matrix=R_matrix.*LineLength;
      | L_matrix=L_matrix.*LineLength;
      | C_matrix=C_matrix.*LineLength;
      | Rg_matrix=Rg_matrix./LineLength;
      | 
      | % Rloss=1/(2*pi*Frequency*C_matrix(1,1)*TangLoss);
      | % Inducdance matrix is slightly modified
      | % beacause the "Mutual Inductance" block does not accept
      | % mutual inductances  equal to self inductances
      | % Diagonal values are multiplied by 1.001
      | nconductors=size(L_matrix,1);
      | for icond=1:nconductors
      |     L_matrix(icond,icond)=L_matrix(icond,icond)*1.001;  
      | end
      mask Display:
      | port_label('lconn',1,'A');
      | port_label('lconn',2,'B');
      | port_label('lconn',3,'C');
      | 
      | port_label('rconn',1,'a');
      | port_label('rconn',2,'b');
      | port_label('rconn',3,'c');
      | 
      | disp('1x240');
  a : PMIOPort  Side=Right
  b : PMIOPort  Port=2  Side=Right
  c : PMIOPort  Port=3  Side=Right
  A : PMIOPort  Port=4  Side=Left
  B : PMIOPort  Port=5  Side=Left
  C : PMIOPort  Port=6  Side=Left
  connections:
  A/RConn1 -- Pi/LConn1 -- DPL/LConn1 -- concentrated/LConn1
  C/RConn1 -- Pi/LConn3 -- concentrated/LConn3 -- DPL/LConn3
  concentrated/RConn2 -- Pi/RConn2 -- Q/LConn2 -- DPL/RConn2
  concentrated/RConn1 -- Pi/RConn1 -- Q/LConn1 -- DPL/RConn1
  concentrated/RConn3 -- Pi/RConn3 -- Q/LConn3 -- DPL/RConn3
  B/RConn1 -- Pi/LConn2 -- DPL/LConn2 -- concentrated/LConn2
  Q/RConn2 -- b/RConn1
  Q/RConn1 -- a/RConn1
  Q/RConn3 -- c/RConn1

== system SPGF_FSK_0000_R2022b/W12 ==
  DPL : Subsystem  Commented=on  mask{N=6, Frequency=[50], R_matrix=[0.347601410823579 0.0494303286168989 0.0494305228057156 0.0494305228057156 0.0494305228057156 0.0494305228057156;0.0494303286168989 0.63357380919679 0.0494305228057156 0.0494305228057156 0.0494305228057156 0.0494305228057156;0.0494305228057156 0.0494305228057156 0.347602052073771 0.0494309698670905 0.0494311641268522 0.0494311641268522;0.0494305228057156 0.0494305228057156 0.0494309698670905 0.633574450446981 0.0494311641268522 0.0494311641268522;0.0494305228057156 0.0494305228057156 0.0494311641268522 0.0494311641268522 0.347602052073771 0.0494309698670905;0.0494305228057156 0.0494305228057156 0.0494311641268522 0.0494311641268522 0.0494309698670905 0.633574450446981], L_matrix=[0.00260859879857304 0.00242332383525137 0.00221745883616686 0.00221745883616686 0.00221745883616686 0.00221745883616686;0.00242332383525137 0.00242198857850016 0.00221745883616686 0.00221745883616686 0.00221745883616686 0.00221745883616686;0.00221745883616686 0.00221745883616686 0.00253519514382882 0.00234992018050715 0.00223977112704788 0.00223977112704788;0.00221745883616686 0.00221745883616686 0.00234992018050715 0.00234858492375594 0.00223977112704788 0.00223977112704788;0.00221745883616686 0.00221745883616686 0.00223977112704788 0.00223977112704788 0.00253519514382882 0.00234992018050715;0.00221745883616686 0.00221745883616686 0.00223977112704788 0.00223977112704788 0.00234992018050715 0.00234858492375594], C_matrix=[1.90757475136094e-07 -1.90757475136094e-07 0 0 0 0;-1.90757475136094e-07 3.66052807704686e-07 0 0 0 0;0 0 1.90757475136094e-07 -1.90757475136094e-07 0 0;0 0 -1.90757475136094e-07 3.66052807704686e-07 0 0;0 0 0 0 1.90757475136094e-07 -1.90757475136094e-07;0 0 0 0 -1.90757475136094e-07 3.66052807704686e-07], Rg_matrix=[834331.357019417 -834331.357019417 Inf Inf Inf -Inf;-834331.357019417 434786.838789375 Inf Inf Inf -Inf;Inf Inf 834331.357019417 -834331.357019417 Inf -Inf;Inf Inf -834331.357019417 434786.838789375 Inf -Inf;Inf Inf Inf Inf 834331.357019417 -834331.357019417;Inf Inf Inf Inf -834331.357019417 434786.838789375], LineLength=[1.5]}
      mask prompts: N "Number of phases [N]"; Frequency "Frequency used for rlc specification [Hz]:"; R_matrix "Resistance per unit length [Ohms/km] NxN matrix"; L_matrix "Inductance per unit length [H/km] NxN matrix"; C_matrix "Capacitance per unit length [F/km] NxN matrix"; Rg_matrix "Resistance shunt matrix 6*6 [Ohm*km]"; LineLength "Line Length(km)"
      mask init:
      | % Rloss=1/(2*pi*Frequency*C_matrix(1,1)*TangLoss);
      | Rg_matrix=Rg_matrix./LineLength;
      mask Display:
      | port_label('lconn',1,'A');
      | port_label('lconn',2,'B');
      | port_label('lconn',3,'C');
      | 
      | port_label('rconn',1,'a');
      | port_label('rconn',2,'b');
      | port_label('rconn',3,'c');
      | 
      | disp('1x95');
  Pi : Subsystem  mask{R0=0.31, X0=0.083, Cp0=0.35, tg=2, Frequency=[50], LineLength=[1.5]}
      mask prompts: R0 "Удельное активное сопротивление, Ом/км"; X0 "Удельное индуктивное сопротивление, Ом/км"; Cp0 "Удельная рабочая емкость, мкФ/км"; tg "Тангенс диэлектрических потерь, %"; Frequency "Частота сети, Гц"; LineLength "Длина линии, км"
      mask init:
      | R=R0*LineLength;
      | L=X0*LineLength/(2*pi*Frequency);
      | Cp=Cp0*LineLength*1e-6;
      | Cmf=0.1525*Cp;
      | Cfg=0.56*Cp;
      | tg_pu=tg/100;
      | 
      | Rmf=1/(Cmf*2*pi*Frequency*tg_pu);
      | Rfg=1/(Cfg*2*pi*Frequency*tg_pu);
      mask Display:
      | port_label('lconn',1,'A');
      | port_label('lconn',2,'B');
      | port_label('lconn',3,'C');
      | 
      | port_label('rconn',1,'a');
      | port_label('rconn',2,'b');
      | port_label('rconn',3,'c');
      | 
      | disp('1x95');
  Q : Subsystem
  concentrated : Subsystem  Commented=on  mask{N=6, Frequency=[50], R_matrix=[0.347601410823579 0.0494303286168989 0.0494305228057156 0.0494305228057156 0.0494305228057156 0.0494305228057156;0.0494303286168989 0.63357380919679 0.0494305228057156 0.0494305228057156 0.0494305228057156 0.0494305228057156;0.0494305228057156 0.0494305228057156 0.347602052073771 0.0494309698670905 0.0494311641268522 0.0494311641268522;0.0494305228057156 0.0494305228057156 0.0494309698670905 0.633574450446981 0.0494311641268522 0.0494311641268522;0.0494305228057156 0.0494305228057156 0.0494311641268522 0.0494311641268522 0.347602052073771 0.0494309698670905;0.0494305228057156 0.0494305228057156 0.0494311641268522 0.0494311641268522 0.0494309698670905 0.633574450446981], L_matrix=[0.00260859879857304 0.00242332383525137 0.00221745883616686 0.00221745883616686 0.00221745883616686 0.00221745883616686;0.00242332383525137 0.00242198857850016 0.00221745883616686 0.00221745883616686 0.00221745883616686 0.00221745883616686;0.00221745883616686 0.00221745883616686 0.00253519514382882 0.00234992018050715 0.00223977112704788 0.00223977112704788;0.00221745883616686 0.00221745883616686 0.00234992018050715 0.00234858492375594 0.00223977112704788 0.00223977112704788;0.00221745883616686 0.00221745883616686 0.00223977112704788 0.00223977112704788 0.00253519514382882 0.00234992018050715;0.00221745883616686 0.00221745883616686 0.00223977112704788 0.00223977112704788 0.00234992018050715 0.00234858492375594], C_matrix=[1.90757475136094e-07 -1.90757475136094e-07 0 0 0 0;-1.90757475136094e-07 3.66052807704686e-07 0 0 0 0;0 0 1.90757475136094e-07 -1.90757475136094e-07 0 0;0 0 -1.90757475136094e-07 3.66052807704686e-07 0 0;0 0 0 0 1.90757475136094e-07 -1.90757475136094e-07;0 0 0 0 -1.90757475136094e-07 3.66052807704686e-07], Rg_matrix=[834331.357019417 -834331.357019417 Inf Inf Inf -Inf;-834331.357019417 434786.838789375 Inf Inf Inf -Inf;Inf Inf 834331.357019417 -834331.357019417 Inf -Inf;Inf Inf -834331.357019417 434786.838789375 Inf -Inf;Inf Inf Inf Inf 834331.357019417 -834331.357019417;Inf Inf Inf Inf -834331.357019417 434786.838789375], LineLength=[1.5]}
      mask prompts: N "Number of phases [N]"; Frequency "Frequency [Hz]:"; R_matrix "Resistance matrix 6*6 [Ohm/km]"; L_matrix "Inductance matrix 6*6 [H/km]"; C_matrix "Capacitance matrix 6*6 [F/km]"; Rg_matrix "Resistance shunt matrix 6*6 [Ohm*km]"; LineLength "Line Length(km)"
      mask init: same as SPGF_FSK_0000_R2022b/W11/concentrated
      mask Display:
      | port_label('lconn',1,'A');
      | port_label('lconn',2,'B');
      | port_label('lconn',3,'C');
      | 
      | port_label('rconn',1,'a');
      | port_label('rconn',2,'b');
      | port_label('rconn',3,'c');
      | 
      | disp('1x95');
  a : PMIOPort  Side=Right
  b : PMIOPort  Port=2  Side=Right
  c : PMIOPort  Port=3  Side=Right
  A : PMIOPort  Port=4  Side=Left
  B : PMIOPort  Port=5  Side=Left
  C : PMIOPort  Port=6  Side=Left
  connections:
  A/RConn1 -- Pi/LConn1 -- concentrated/LConn1 -- DPL/LConn1
  C/RConn1 -- Pi/LConn3 -- concentrated/LConn3 -- DPL/LConn3
  Pi/RConn2 -- Q/LConn2 -- concentrated/RConn2 -- DPL/RConn2
  Pi/RConn1 -- Q/LConn1 -- concentrated/RConn1 -- DPL/RConn1
  Pi/RConn3 -- Q/LConn3 -- concentrated/RConn3 -- DPL/RConn3
  B/RConn1 -- Pi/LConn2 -- concentrated/LConn2 -- DPL/LConn2
  Q/RConn2 -- b/RConn1
  Q/RConn1 -- a/RConn1
  Q/RConn3 -- c/RConn1

== system SPGF_FSK_0000_R2022b/W13 ==
  DPL : Subsystem  Commented=on  mask{N=6, Frequency=[50], R_matrix=[0.347601410823579 0.0494303286168989 0.0494305228057156 0.0494305228057156 0.0494305228057156 0.0494305228057156;0.0494303286168989 0.63357380919679 0.0494305228057156 0.0494305228057156 0.0494305228057156 0.0494305228057156;0.0494305228057156 0.0494305228057156 0.347602052073771 0.0494309698670905 0.0494311641268522 0.0494311641268522;0.0494305228057156 0.0494305228057156 0.0494309698670905 0.633574450446981 0.0494311641268522 0.0494311641268522;0.0494305228057156 0.0494305228057156 0.0494311641268522 0.0494311641268522 0.347602052073771 0.0494309698670905;0.0494305228057156 0.0494305228057156 0.0494311641268522 0.0494311641268522 0.0494309698670905 0.633574450446981], L_matrix=[0.00260859879857304 0.00242332383525137 0.00221745883616686 0.00221745883616686 0.00221745883616686 0.00221745883616686;0.00242332383525137 0.00242198857850016 0.00221745883616686 0.00221745883616686 0.00221745883616686 0.00221745883616686;0.00221745883616686 0.00221745883616686 0.00253519514382882 0.00234992018050715 0.00223977112704788 0.00223977112704788;0.00221745883616686 0.00221745883616686 0.00234992018050715 0.00234858492375594 0.00223977112704788 0.00223977112704788;0.00221745883616686 0.00221745883616686 0.00223977112704788 0.00223977112704788 0.00253519514382882 0.00234992018050715;0.00221745883616686 0.00221745883616686 0.00223977112704788 0.00223977112704788 0.00234992018050715 0.00234858492375594], C_matrix=[1.90757475136094e-07 -1.90757475136094e-07 0 0 0 0;-1.90757475136094e-07 3.66052807704686e-07 0 0 0 0;0 0 1.90757475136094e-07 -1.90757475136094e-07 0 0;0 0 -1.90757475136094e-07 3.66052807704686e-07 0 0;0 0 0 0 1.90757475136094e-07 -1.90757475136094e-07;0 0 0 0 -1.90757475136094e-07 3.66052807704686e-07], Rg_matrix=[834331.357019417 -834331.357019417 Inf Inf Inf -Inf;-834331.357019417 434786.838789375 Inf Inf Inf -Inf;Inf Inf 834331.357019417 -834331.357019417 Inf -Inf;Inf Inf -834331.357019417 434786.838789375 Inf -Inf;Inf Inf Inf Inf 834331.357019417 -834331.357019417;Inf Inf Inf Inf -834331.357019417 434786.838789375], LineLength=[2.3]}
      mask prompts: N "Number of phases [N]"; Frequency "Frequency used for rlc specification [Hz]:"; R_matrix "Resistance per unit length [Ohms/km] NxN matrix"; L_matrix "Inductance per unit length [H/km] NxN matrix"; C_matrix "Capacitance per unit length [F/km] NxN matrix"; Rg_matrix "Resistance shunt matrix 6*6 [Ohm*km]"; LineLength "Line Length(km)"
      mask init:
      | % Rloss=1/(2*pi*Frequency*C_matrix(1,1)*TangLoss);
      | Rg_matrix=Rg_matrix./LineLength;
      mask Display:
      | port_label('lconn',1,'A');
      | port_label('lconn',2,'B');
      | port_label('lconn',3,'C');
      | 
      | port_label('rconn',1,'a');
      | port_label('rconn',2,'b');
      | port_label('rconn',3,'c');
      | 
      | disp('1x95');
  Pi : Subsystem  mask{R0=0.31, X0=0.083, Cp0=0.35, tg=2, Frequency=[50], LineLength=[2.3]}
      mask prompts: R0 "Удельное активное сопротивление, Ом/км"; X0 "Удельное индуктивное сопротивление, Ом/км"; Cp0 "Удельная рабочая емкость, мкФ/км"; tg "Тангенс диэлектрических потерь, %"; Frequency "Частота сети, Гц"; LineLength "Длина линии, км"
      mask init:
      | R=R0*LineLength;
      | L=X0*LineLength/(2*pi*Frequency);
      | Cp=Cp0*LineLength*1e-6;
      | Cmf=0.1525*Cp;
      | Cfg=0.56*Cp;
      | tg_pu=tg/100;
      | 
      | Rmf=1/(Cmf*2*pi*Frequency*tg_pu);
      | Rfg=1/(Cfg*2*pi*Frequency*tg_pu);
      mask Display:
      | port_label('lconn',1,'A');
      | port_label('lconn',2,'B');
      | port_label('lconn',3,'C');
      | 
      | port_label('rconn',1,'a');
      | port_label('rconn',2,'b');
      | port_label('rconn',3,'c');
      | 
      | disp('1x95');
  Q : Subsystem
  concentrated : Subsystem  Commented=on  mask{N=6, Frequency=[50], R_matrix=[0.347601410823579 0.0494303286168989 0.0494305228057156 0.0494305228057156 0.0494305228057156 0.0494305228057156;0.0494303286168989 0.63357380919679 0.0494305228057156 0.0494305228057156 0.0494305228057156 0.0494305228057156;0.0494305228057156 0.0494305228057156 0.347602052073771 0.0494309698670905 0.0494311641268522 0.0494311641268522;0.0494305228057156 0.0494305228057156 0.0494309698670905 0.633574450446981 0.0494311641268522 0.0494311641268522;0.0494305228057156 0.0494305228057156 0.0494311641268522 0.0494311641268522 0.347602052073771 0.0494309698670905;0.0494305228057156 0.0494305228057156 0.0494311641268522 0.0494311641268522 0.0494309698670905 0.633574450446981], L_matrix=[0.00260859879857304 0.00242332383525137 0.00221745883616686 0.00221745883616686 0.00221745883616686 0.00221745883616686;0.00242332383525137 0.00242198857850016 0.00221745883616686 0.00221745883616686 0.00221745883616686 0.00221745883616686;0.00221745883616686 0.00221745883616686 0.00253519514382882 0.00234992018050715 0.00223977112704788 0.00223977112704788;0.00221745883616686 0.00221745883616686 0.00234992018050715 0.00234858492375594 0.00223977112704788 0.00223977112704788;0.00221745883616686 0.00221745883616686 0.00223977112704788 0.00223977112704788 0.00253519514382882 0.00234992018050715;0.00221745883616686 0.00221745883616686 0.00223977112704788 0.00223977112704788 0.00234992018050715 0.00234858492375594], C_matrix=[1.90757475136094e-07 -1.90757475136094e-07 0 0 0 0;-1.90757475136094e-07 3.66052807704686e-07 0 0 0 0;0 0 1.90757475136094e-07 -1.90757475136094e-07 0 0;0 0 -1.90757475136094e-07 3.66052807704686e-07 0 0;0 0 0 0 1.90757475136094e-07 -1.90757475136094e-07;0 0 0 0 -1.90757475136094e-07 3.66052807704686e-07], Rg_matrix=[834331.357019417 -834331.357019417 Inf Inf Inf -Inf;-834331.357019417 434786.838789375 Inf Inf Inf -Inf;Inf Inf 834331.357019417 -834331.357019417 Inf -Inf;Inf Inf -834331.357019417 434786.838789375 Inf -Inf;Inf Inf Inf Inf 834331.357019417 -834331.357019417;Inf Inf Inf Inf -834331.357019417 434786.838789375], LineLength=[2.3]}
      mask prompts: N "Number of phases [N]"; Frequency "Frequency [Hz]:"; R_matrix "Resistance matrix 6*6 [Ohm/km]"; L_matrix "Inductance matrix 6*6 [H/km]"; C_matrix "Capacitance matrix 6*6 [F/km]"; Rg_matrix "Resistance shunt matrix 6*6 [Ohm*km]"; LineLength "Line Length(km)"
      mask init: same as SPGF_FSK_0000_R2022b/W11/concentrated
      mask Display:
      | port_label('lconn',1,'A');
      | port_label('lconn',2,'B');
      | port_label('lconn',3,'C');
      | 
      | port_label('rconn',1,'a');
      | port_label('rconn',2,'b');
      | port_label('rconn',3,'c');
      | 
      | disp('1x95');
  a : PMIOPort  Side=Right
  b : PMIOPort  Port=2  Side=Right
  c : PMIOPort  Port=3  Side=Right
  A : PMIOPort  Port=4  Side=Left
  B : PMIOPort  Port=5  Side=Left
  C : PMIOPort  Port=6  Side=Left
  connections:
  Q/RConn3 -- c/RConn1
  Q/RConn1 -- a/RConn1
  Q/RConn2 -- b/RConn1
  Pi/LConn2 -- DPL/LConn2 -- concentrated/LConn2 -- B/RConn1
  Pi/RConn3 -- Q/LConn3 -- DPL/RConn3 -- concentrated/RConn3
  Pi/RConn1 -- Q/LConn1 -- DPL/RConn1 -- concentrated/RConn1
  Pi/RConn2 -- Q/LConn2 -- DPL/RConn2 -- concentrated/RConn2
  Pi/LConn3 -- concentrated/LConn3 -- DPL/LConn3 -- C/RConn1
  Pi/LConn1 -- DPL/LConn1 -- concentrated/LConn1 -- A/RConn1
